simulink model "PASTASimulation"  (R2014a)
settings: Solver=FixedStepDiscrete  StartTime=0.0  StopTime=Inf  FixedStep=1  RelTol=1e-3
InitFcn:
  | Set_Sensor_Priorities
StartFcn:
  | Initialize
values from neighbouring files (symbols this model uses):
  hum_st = pri_hum_st+1    (= 2)    [Set_Sensor_Priorities.m]    (also in humid_rand_gen.m = evalin('base','hum_st'))
  press_st = pri_press_st+1    (= 4)    [Set_Sensor_Priorities.m]    (also in press_rand_gen.m = evalin('base','press_st'))
  temp_st = pri_temp_st+1    (= 3)    [Set_Sensor_Priorities.m]    (also in temp_rand_gen.m = evalin('base','temp_st'))
  wind_st = pri_wind_st+1    (= 5)    [Set_Sensor_Priorities.m]    (also in wind_rand_gen.m = evalin('base','wind_st'))
undefined symbols (not defined in the file or in its folder): humid_rand_gen, press_rand_gen, temp_rand_gen, wind_rand_gen
libraries: realtime_pacer_lib x1
settings Model: Creator=Aditya  LastModifiedBy=Aditya
settings DebuggingCC: SignalResolutionControl=TryResolveAllWithWarning  InheritedTsInSrcMsg=none  MultiTaskRateTransMsg=warning  UniqueDataStoreMsg=warning

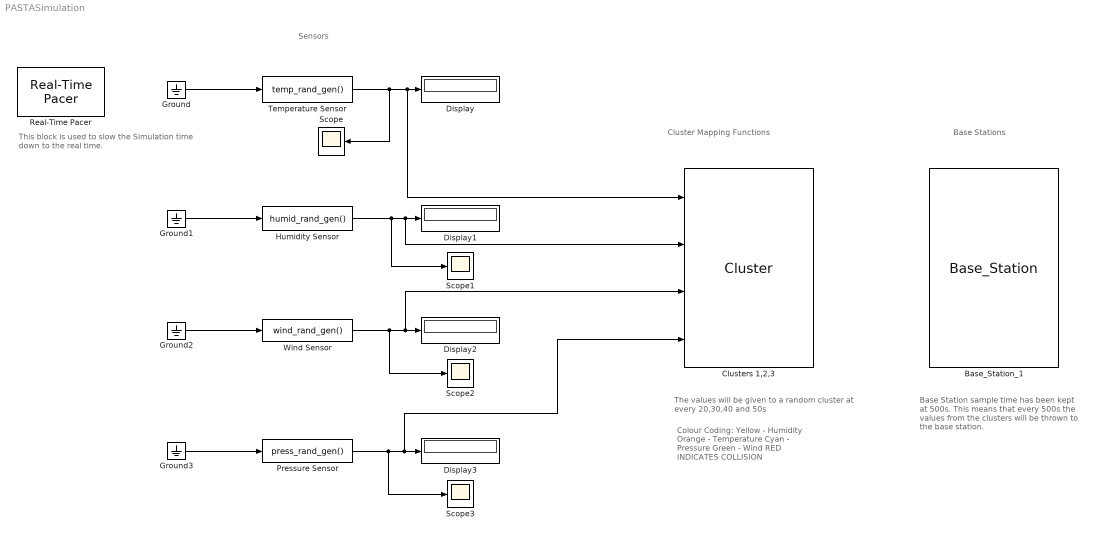
== system PASTASimulation ==
  note: Colour Coding:
      | Yellow - Humidity
      | Orange - Temperature
      | Cyan - Pressure
      | Green - Wind
      | RED INDICATES COLLISION
  note: This block is used to slow the Simulation
      | time down to the real time.
  note: Base Station sample time has been
      | kept at 500s. This means that every
      | 500s the values from the clusters will
      | be thrown to the base station.
  note: Sensors
  note: Cluster Mapping Functions
  note: Base Stations
  note: The values will be given to a random cluster
      | at every 20,30,40 and 50s
  Base_Station_1 : M-S-Function  FunctionName=Base_Station
      mask Display:
      | % port_label('input',1,'Temperature')
      | % port_label('input',2,'Humidity')
      | % port_label('input',3,'Wind')
      | % port_label('input',4,'Pressure')
      | fprintf('Base Station')
  Clusters 1,2,3 : M-S-Function  FunctionName=Cluster
      mask Display:
      | port_label('input',1,'Temperature')
      | port_label('input',2,'Humidity')
      | port_label('input',3,'Wind')
      | port_label('input',4,'Pressure')
      | fprintf('Clusters')
  Display{,1..3} (4 alike) : Display
  Ground{,1..3} (4 alike) : Ground
  Humidity Sensor : MATLABFcn  MATLABFcn=humid_rand_gen()  SampleTime=hum_st
      mask Display: fprintf('Humidity Sensor')
  Pressure Sensor : MATLABFcn  MATLABFcn=press_rand_gen()  SampleTime=press_st
      mask Display: fprintf('Pressure Sensor')
  Real-Time Pacer : realtime_pacer_lib/Real-Time Pacer  simTimePerRealTime=150
  Scope{,1..3} (4 alike) : Scope
      Scope settings: YMin=-50  YMax=120
      Scope1 settings: YMin=57.5  YMax=90
      Scope2 settings: SaveName=ScopeData2
      Scope3 settings: SaveName=ScopeData3
  Temperature Sensor : MATLABFcn  MATLABFcn=temp_rand_gen()  SampleTime=temp_st
      mask Display: fprintf('Temperature Sensor')
  Wind Sensor : MATLABFcn  MATLABFcn=wind_rand_gen()  SampleTime=wind_st
      mask Display: fprintf('Wind Sensor')
  wires:
  Temperature Sensor/1 -> Scope/1, Clusters 1,2,3/1, Display/1
  Ground/1 -> Temperature Sensor/1
  Humidity Sensor/1 -> Scope1/1, Clusters 1,2,3/2, Display1/1
  Ground1/1 -> Humidity Sensor/1
  Wind Sensor/1 -> Scope2/1, Clusters 1,2,3/3, Display2/1
  Ground2/1 -> Wind Sensor/1
  Pressure Sensor/1 -> Scope3/1, Clusters 1,2,3/4, Display3/1
  Ground3/1 -> Pressure Sensor/1
